simulink model "Copy_of_htx_estimator"  (R2024b)
settings: Solver=FixedStepAuto  StartTime=0.0  StopTime=10.0  RelTol=1e-3
undefined symbols (not defined in the file): dspblkCoreblockFVToolHelper, gcbh
libraries: simulink_extras x1
settings Model: Creator=lukec  LastModifiedBy=lukec
settings OptimizationCC: DefaultParameterBehavior=Inlined  EnhancedBackFolding=on  PassReuseOutputArgsAs=Individual arguments  ZeroExternalMemoryAtStartup=off  ZeroInternalMemoryAtStartup=off  OptimizeBlockOrder=speed  DifferentSizesBufferReuse=on  OptimizationCustomize=off  EfficientTunableParamExpr=on
settings DebuggingCC: ParameterTunabilityLossMsg=error
settings HardwareCC: ProdBitPerPointer=32  ProdBitPerSizeT=32  ProdBitPerPtrDiffT=32  ProdLargestAtomicInteger=Long  ProdLargestAtomicFloat=Double  ProdWordSize=32  ProdHWDeviceType=ARM Compatible->ARM Cortex-M
settings SFSimCC: MATLABDynamicMemAlloc=off
settings RTWCC: Description=Embedded Coder  SystemTargetFile=ert.tlc  GenCodeOnly=on  PackageGeneratedCodeAndArtifacts=on  TemplateMakefile=ert_default_tmf  Toolchain=CMake  TargetLang=C++
settings CodeAppCC: ForceParamTrailComments=on  IgnoreCustomStorageClasses=off  MaxIdLength=255  OperatorAnnotations=on  SimulinkDataObjDesc=on  SFDataObjDesc=on  InsertBlockDesc=on
settings ERTTargetCC: TargetLangStandard=C++17 (ISO)  CodeInterfacePackaging=C++ class  RootIOFormat=Structure reference  ERTCustomFileTemplate=example_file_process.tlc  ArrayContainerType=std::array

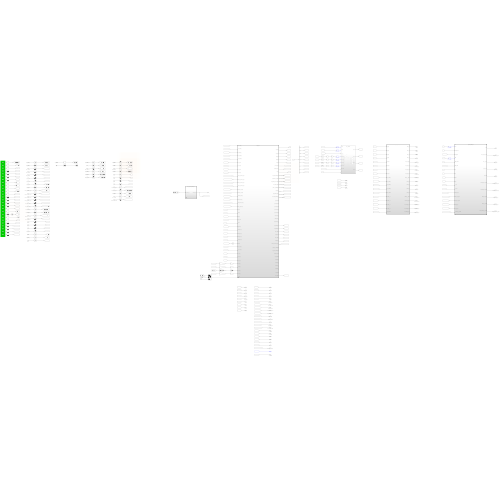
[thumbnail: Simulink's stored preview of the top-level diagram]
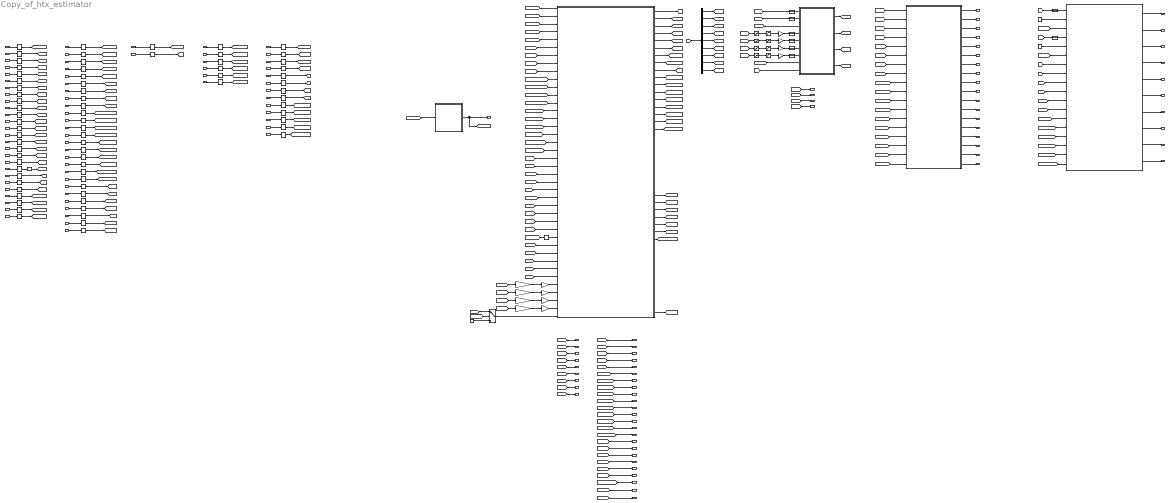
== system Copy_of_htx_estimator ==
  note: non-param-inputs
  steer_sensor_raw : Inport
  ax_m_s2 : Inport  Port=2
  ay_m_s2 : Inport  Port=3
  loadcell_fl : Inport  Port=4
  loadcell_fr : Inport  Port=5
  loadcell_rl : Inport  Port=6
  loadcell_rr : Inport  Port=7
  torq_Nm_fl : Inport  Port=8
  torq_Nm_fr : Inport  Port=9
  torq_Nm_rl : Inport  Port=10
  torq_Nm_rr : Inport  Port=11
  motor_rpm_fl : Inport  Port=12
  motor_rpm_fr : Inport  Port=13
  motor_rpm_rl : Inport  Port=14
  motor_rpm_rr : Inport  Port=15
  vx_raw_m_s : Inport  Port=16
  vy_raw_m_s : Inport  Port=17
  ins_vel_u : Inport  Port=18
  ins_mode : Inport  Port=19
  accel : Inport  Port=20
  brake : Inport  Port=21
  wz_rad_s : Inport  Port=22
  motor_temp_C_fl : Inport  Port=23
  motor_temp_C_fr : Inport  Port=24
  motor_temp_C_rl : Inport  Port=25
  motor_temp_C_rr : Inport  Port=26
  proc_vx_std_m_s : Inport  Port=27
  proc_vy_std_m_s : Inport  Port=28
  proc_r_std_deg_s : Inport  Port=29
  proc_ax_std_m_s2 : Inport  Port=30
  proc_ay_std_m_s2 : Inport  Port=31
  proc_sr_fl_std : Inport  Port=32
  proc_sr_fr_std : Inport  Port=33
  proc_sr_rl_std : Inport  Port=34
  proc_sr_rr_std : Inport  Port=35
  meas_ins_vx_mode1_std_m_s : Inport  Port=36
  meas_ins_vy_mode1_std_m_s : Inport  Port=37
  meas_ins_vx_mode2_std_m_s : Inport  Port=38
  meas_ins_vy_mode2_std_m_s : Inport  Port=39
  meas_imu_ax_std_m_s2 : Inport  Port=40
  meas_imu_ay_std_m_s2 : Inport  Port=41
  meas_imu_r_std_deg_s : Inport  Port=42
  meas_wss_std_deg_s : Inport  Port=43
  meas_pseudo_vx_std_m_s : Inport  Port=44
  meas_vy_gate_std_m_s : Inport  Port=45
  chi_ins_vx : Inport  Port=46
  chi_ins_vy : Inport  Port=47
  chi_imu_r : Inport  Port=48
  chi_imu_accel : Inport  Port=49
  chi_wss : Inport  Port=50
  chi_pseudo_vx : Inport  Port=51
  fz_meas_alpha : Inport  Port=52
  m_kg : Inport  Port=53
  amk_eff_modifier_fl : Inport  Port=54
  amk_eff_modifier_fr : Inport  Port=55
  amk_eff_modifier_rl : Inport  Port=56
  amk_eff_modifier_rr : Inport  Port=57
  global_eff_modifier : Inport  Port=58
  brake_eff_modifier : Inport  Port=59
  accel_deadzone : Inport  Port=60
  accel_gamma : Inport  Port=61
  brake_deadzone : Inport  Port=62
  brake_gamma : Inport  Port=63
  a_off : Inport  Port=64
  a_on : Inport  Port=65
  b_start : Inport  Port=66
  b_full : Inport  Port=67
  drive_motor_torq_lim : Inport  Port=68
  regen_motor_torq_lim : Inport  Port=69
  motor_rpm_lim : Inport  Port=70
  elec_p_lim_kW : Inport  Port=71
  per_motor_elec_p_lim_kW : Inport  Port=72
  use_ins : Inport  Port=73
  1-D Lookup Table : Lookup_n-D  NumberOfTableDimensions=1  BreakpointsForDimension1=|  Table=|  ExtrapMethod=Clip  InternalRulePriority=Speed  RndMeth=Simplest
      BreakpointsForDimension1=|
      | [159
      | 845
      | 1004
      | 1093
      | 1233
      | 1645
      | 1875
      | 2150
      | 2260]
      Table=|
      | [0
      | 87.3
      | 107.7
      | 120.1
      | 139.7
      | 193.3
      | 230.4
      | 269.1
      | 282.5]
  1-D Lookup Table1 : Lookup_n-D  NumberOfTableDimensions=1  BreakpointsForDimension1=|  Table=|  ExtrapMethod=Clip  InternalRulePriority=Speed  RndMeth=Simplest
      BreakpointsForDimension1=|
      | [191
      | 984
      | 1101
      | 1186
      | 1323
      | 1730
      | 1962
      | 2150
      | 2350
      | ]
      Table=|
      | [0
      | 102.4
      | 116.4
      | 128.2
      | 148.6
      | 198.5
      | 236.2
      | 260.2
      | 289.2
      | ]
  1-D Lookup Table2 : Lookup_n-D  NumberOfTableDimensions=1  BreakpointsForDimension1=|  Table=|  ExtrapMethod=Clip  InternalRulePriority=Speed  RndMeth=Simplest
      BreakpointsForDimension1=|
      | [223
      | 1017
      | 1069
      | 1193
      | 1260
      | 1730
      | 1992
      | 2170
      | 2310
      | ]
      Table=|
      | [0
      | 112.9
      | 117.6
      | 135.2
      | 146.8
      | 213.3
      | 250.6
      | 276.9
      | 296.5
      | ]
  1-D Lookup Table3 : Lookup_n-D  NumberOfTableDimensions=1  BreakpointsForDimension1=|  Table=|  ExtrapMethod=Clip  InternalRulePriority=Speed  RndMeth=Simplest
      BreakpointsForDimension1=|
      | [219
      | 908
      | 1006
      | 1134
      | 1180
      | 1685
      | 1935
      | 2093
      | 2240
      | ]
      Table=|
      | [0
      | 98.9
      | 110.4
      | 128.8
      | 137.2
      | 209.7
      | 242.8
      | 268.2
      | 288.5
      | ]
  Constant : Constant  Value=0
  Constant1 : Constant  Value=0
  Constant2 : Constant  Value=0
  Degrees to Radians : simulink_extras/Transformations/Degrees to Radians
  Demux : Demux  Outputs=9
  Floor : Rounding
  Gain{,2,4,6} (4 alike) : Gain  Gain=0.1047197551196598
  Gain{1,3,5,7} (4 alike) : Gain  Gain=1/11.83
  Gain{8..11} (4 alike) : Gain  Gain=4.4482
  Model : ModelReference  ModelNameDialog=htx_wheel_steer_estimator_base.slx  SimulationMode=Normal  ModelReferenceVersion=1.9
  Model1 : ModelReference  ModelNameDialog=htx_amk_eff_estimator_base.slx  SimulationMode=Normal  ModelReferenceVersion=1.36
  Model2 : ModelReference  ModelNameDialog=htx_intent_estimator_base.slx  SimulationMode=Normal  ModelReferenceVersion=1.15
  Model6 : ModelReference  ModelNameDialog=htx_ekf_base.slx  SimulationMode=Normal  ModelReferenceVersion=1.26
      settings: PortSchema="{\"entries\":[{\"content\":{\"sides\":[{\"content\":{\"connectorIds\":[\"In1\",\"In2\",\"In3\",\"In4\",\"In5\",\"In6\",\"In7\",\"In8\",\"In9\",\"In10\",\"In11\",\"In12\",\"In13\",\"In14\",\"In15\",\"In16\",\"In17\",\"In18\",\"In19\",\"In20\",\"In21\",\"In22\",\"In23\",\"In24\",\"In40\",\"In25\",\"In26\",\"In27\",\"In28\",\"In29\",\"In30\",\"In31\",\"In32\",\"In33\",\"In34\",\"In35\",\"In36\",\"In37\",\"In38\",\"In39\"]},\"type\":\"ConnectorPlacement.EquallySpacedRectSide\",\"uuid\":\"bb5109ea-6939-45c2-a357-a710596eeb4b\"},{\"content\":{\"connectorIds\":[\"Out1\",\"Out2\",\"Out3\",\"Out4\",\"Out5\",\"Out6\",\"Out7\",\"Out8\",\"Out9\",\"Out10\",\"Out11\",\"Out12\",\"Out13\",\"Out14\",\"Out15\",\"Out16\",\"Out17\",\"Out18\",\"Out19\",\"Out20\",\"Out21\",\"Out22\",\"Out23\",\"Out24\",\"Out25\",\"Out26\",\"Out27\",\"Out28\",\"Out29\",\"Out30\",\"Out31\",\"Out32\",\"Out33\",\"Out34\",\"Out35\",\"Out36\",\"Out37\",\"Out38\",\"Out39\",\"Out40\",\"Out41\",\"Out42\"],\"side\":\"RIGHT\"},\"type\":\"ConnectorPlacement.EquallySpacedRectSide\",\"uuid\":\"76f86590-693a-4540-9c0b-c0cd03bb8a5c\"},{\"content\":{\"side\":\"TOP\"},\"type\":\"ConnectorPlacement.EquallySpacedRectSide\",\"uuid\":\"14cceb79-494c-4b5e-a97a-eec243580695\"}]},\"type\":\"ConnectorPlacement.EquallySpacedConnector\",\"uuid\":\"129f1803-a8f8-4413-b20a-49775fdc7b41\"}],\"packageUris\":[\"http://schema.mathworks.com/mf0/Connector/R2020b\"],\"version\":\"1.0\"}"
  Rate Transition{,1..72} (73 alike) : RateTransition  OutPortSampleTime=0.004
  Saturation{,1..3} (4 alike) : Saturate  UpperLimit=350  LowerLimit=0
  Subsystem : Subsystem  ReferencedSubsystem=htx_fz_estimator
  Switch : Switch  Criteria=u2 > Threshold  SaturateOnIntegerOverflow=off  InputSameDT=off
  low-pass_0.035 {1..8} (8 alike) : DiscreteTransferFcn  LoadFcn=dspblkCoreblockFVToolHelper(gcbh,'load');  Numerator=[0, 0.1143]  Denominator=[1, -0.8857]
      settings: CopyFcn=dspblkCoreblockFVToolHelper(gcbh,'copy');  DeleteFcn=dspblkCoreblockFVToolHelper(gcbh,'close');  ModelCloseFcn=dspblkCoreblockFVToolHelper(gcbh,'close');  PreSaveFcn=dspblkCoreblockFVToolHelper(gcbh,'presave');  PostSaveFcn=dspblkCoreblockFVToolHelper(gcbh,'postsave');  CloseFcn=dspblkCoreblockFVToolHelper(gcbh,'close');
  wheel_steer_deg : Outport
  ekf_vx_m_s : Outport  Port=2
  ekf_vy_m_s : Outport  Port=3
  ekf_r_rad_s : Outport  Port=4
  ekf_ax_m_s2 : Outport  Port=5
  ekf_ay_m_s2 : Outport  Port=6
  ekf_sr_fl : Outport  Port=7
  ekf_sr_fr : Outport  Port=8
  ekf_sr_rl : Outport  Port=9
  ekf_sr_rr : Outport  Port=10
  ins_vx_fault : Outport  Port=11
  ins_vy_fault : Outport  Port=12
  imu_r_fault : Outport  Port=13
  imu_a_fault : Outport  Port=14
  wss_fault : Outport  Port=15
  pseudo_vx_fault : Outport  Port=16
  use_pseudo_vx_flag : Outport  Port=17
  ins_supervisor_mode : Outport  Port=18
  ins_supervisor_fail_count : Outport  Port=19
  ins_supervisor_good_count : Outport  Port=20
  ins_reports_valid : Outport  Port=21
  pseudo_vx_available : Outport  Port=22
  use_ins_dbg : Outport  Port=23
  ins_vx_update_used : Outport  Port=24
  ins_low_speed_override : Outport  Port=25
  spin_detected : Outport  Port=26
  lock_detected : Outport  Port=27
  spin_front : Outport  Port=28
  spin_rear : Outport  Port=29
  lock_front : Outport  Port=30
  lock_rear : Outport  Port=31
  decouple_wss_from_vxvy : Outport  Port=32
  fz_est_N_fl : Outport  Port=33
  fz_est_N_fr : Outport  Port=34
  fz_est_N_rl : Outport  Port=35
  fz_est_N_rr : Outport  Port=36
  amk_eff_fl : Outport  Port=37
  amk_eff_fr : Outport  Port=38
  amk_eff_rl : Outport  Port=39
  amk_eff_rr : Outport  Port=40
  amk_elec_p_W_fl : Outport  Port=41
  amk_elec_p_W_fr : Outport  Port=42
  amk_elec_p_W_rl : Outport  Port=43
  amk_elec_p_W_rr : Outport  Port=44
  amk_elec_p_kW_tot : Outport  Port=45
  global_eff_fl : Outport  Port=46
  global_eff_fr : Outport  Port=47
  global_eff_rl : Outport  Port=48
  global_eff_rr : Outport  Port=49
  global_elec_p_kW_tot : Outport  Port=50
  motor_heat_gen_W_fl : Outport  Port=51
  motor_heat_gen_W_fr : Outport  Port=52
  motor_heat_gen_W_rl : Outport  Port=53
  motor_heat_gen_W_rr : Outport  Port=54
  intent : Outport  Port=55
  max_tot_motor_torq_Nm : Outport  Port=56
  des_wz_rad_s : Outport  Port=57
  w_z_error_rad_s : Outport  Port=58
  des_Mz_Nm : Outport  Port=59
  intent_drive_motor_torq_lim : Outport  Port=60
  intent_regen_motor_torq_lim : Outport  Port=61
  intent_motor_rpm_lim : Outport  Port=62
  intent_elec_p_lim_kW : Outport  Port=63
  intent_per_motor_elec_p_lim_kW : Outport  Port=64
  intent_use_ins : Outport  Port=65
  ins_state_dbg : Outport  Port=66
  wires:
  ax_m_s2/1 -> Rate Transition2/1
  motor_temp_C_fl/1 -> Rate Transition1/1
  motor_temp_C_rr/1 -> Rate Transition58/1
  torq_Nm_fr/1 -> Rate Transition9/1
  Rate Transition58/1 -> [motor_temp_C_rr]
  Rate Transition11/1 -> [torq_Nm_rr]
  Rate Transition22/1 -> [accel]
  Rate Transition/1 -> [steer_sensor_raw]
  Rate Transition13/1 -> Floor/1
  vy_raw_m_s/1 -> Rate Transition19/1
  loadcell_rl/1 -> Rate Transition6/1
  ins_vel_u/1 -> Rate Transition12/1
  Rate Transition3/1 -> [imu_ay_m_s2]
  Rate Transition18/1 -> [ins_vx_m_s]
  Rate Transition10/1 -> [torq_Nm_rl]
  Rate Transition4/1 -> [loadcell_fl]
  Rate Transition12/1 -> [ins_vel_u]
  Rate Transition59/1 -> [motor_temp_C_fr]
  motor_temp_C_rl/1 -> Rate Transition57/1
  loadcell_fl/1 -> Rate Transition4/1
  motor_rpm_rr/1 -> Rate Transition17/1
  brake/1 -> Rate Transition20/1
  steer_sensor_raw/1 -> Rate Transition/1
  vx_raw_m_s/1 -> Rate Transition18/1
  Rate Transition14/1 -> [motor_rpm_fl]
  Rate Transition7/1 -> [loadcell_rr]
  wz_rad_s/1 -> Rate Transition21/1
  Rate Transition5/1 -> [loadcell_fr]
  Rate Transition2/1 -> [imu_ax_m_s2]
  ins_mode/1 -> Rate Transition13/1
  Rate Transition17/1 -> [motor_rpm_rr]
  Rate Transition9/1 -> [torq_Nm_fr]
  accel/1 -> Rate Transition22/1
  torq_Nm_rl/1 -> Rate Transition10/1
  Rate Transition6/1 -> [loadcell_rl]
  motor_rpm_rl/1 -> Rate Transition16/1
  motor_rpm_fl/1 -> Rate Transition14/1
  motor_rpm_fr/1 -> Rate Transition15/1
  Rate Transition16/1 -> [motor_rpm_rl]
  Rate Transition19/1 -> [ins_vy_m_s]
  Rate Transition20/1 -> [brake]
  torq_Nm_rr/1 -> Rate Transition11/1
  loadcell_rr/1 -> Rate Transition7/1
  Rate Transition8/1 -> [torq_Nm_fl]
  Rate Transition15/1 -> [motor_rpm_fr]
  Rate Transition57/1 -> [motor_temp_C_rl]
  Rate Transition1/1 -> [motor_temp_C_fl]
  torq_Nm_fl/1 -> Rate Transition8/1
  motor_temp_C_fr/1 -> Rate Transition59/1
  loadcell_fr/1 -> Rate Transition5/1
  ay_m_s2/1 -> Rate Transition3/1
  Rate Transition21/1 -> [imu_r_rad_s]
  [steer_sensor_raw] -> Model/1
  Model/1 -> wheel_steer_deg/1, [wheel_steer_deg]
  low-pass_0.035 5/1 -> Subsystem/1
  [imu_ax_m_s2] -> low-pass_0.035 5/1
  low-pass_0.035 6/1 -> Subsystem/2
  [imu_ay_m_s2] -> low-pass_0.035 6/1
  [loadcell_fr] -> 1-D Lookup Table1/1
  [loadcell_rl] -> 1-D Lookup Table2/1
  [loadcell_rr] -> 1-D Lookup Table3/1
  1-D Lookup Table/1 -> Saturation/1
  low-pass_0.035 3/1 -> Subsystem/4
  1-D Lookup Table1/1 -> Saturation1/1
  low-pass_0.035 2/1 -> Subsystem/6
  low-pass_0.035 4/1 -> Subsystem/7
  low-pass_0.035 1/1 -> Subsystem/5
  1-D Lookup Table2/1 -> Saturation2/1
  1-D Lookup Table3/1 -> Saturation3/1
  Subsystem/1 -> [fz_est_N_fl]
  Subsystem/2 -> [fz_est_N_fr]
  Subsystem/3 -> [fz_est_N_rl]
  Subsystem/4 -> [fz_est_N_rr]
  [torq_Nm_fl] -> Model6/25
  [torq_Nm_fr] -> Model6/26
  [torq_Nm_rl] -> Model6/27
  [torq_Nm_rr] -> Model6/28
  [wheel_steer_deg] -> Degrees to Radians/1
  Degrees to Radians/1 -> Model6/29
  [ins_vx_m_s] -> Model6/30
  [ins_vy_m_s] -> Model6/31
  [imu_r_rad_s] -> Model6/32
  [imu_ax_m_s2] -> Model6/33
  [imu_ay_m_s2] -> Model6/34
  [motor_rpm_fl] -> Gain/1
  Gain/1 -> Gain1/1
  Gain1/1 -> Model6/35
  Gain3/1 -> Model6/36
  [motor_rpm_fr] -> Gain2/1
  [motor_rpm_rl] -> Gain4/1
  Gain5/1 -> Model6/37
  Gain7/1 -> Model6/38
  [motor_rpm_rr] -> Gain6/1
  Model6/1 -> [x]  "x"
  Model6/2 -> [ins_vx_fault]
  Model6/3 -> [ins_vy_fault]
  Model6/4 -> [imu_r_fault]
  Model6/5 -> [imu_a_fault]
  Model6/6 -> [wss_fault]
  Model6/7 -> [pseudo_vx_fault]
  Model6/8 -> [use_pseudo_vx_flag]
  Model6/9 -> [P_diag]
  Model6/10 -> [ins_supervisor_mode]  "ins_supervisor_mode_dbg"
  Model6/11 -> [ins_supervisor_fail_count]  "ins_supervisor_fail_count_dbg"
  Model6/12 -> [ins_supervisor_good_count]  "ins_supervisor_good_count_dbg"
  Model6/13 -> [ins_resports_valid]  "ins_reports_valid_dbg"
  Model6/14 -> [pseudo_vx_available]  "pseudo_vx_available_dbg"
  Model6/15 -> [use_ins_dbg]  "use_ins_dbg"
  Model6/16 -> [ins_vx_update_used]  "ins_vx_update_used_dbg"
  Model6/17 -> [ins_low_speed_override]  "ins_low_speed_override_dbg"
  Model6/26 -> [spin_detected]
  Model6/27 -> [lock_detected]
  Model6/28 -> [spin_front]
  Model6/29 -> [spin_rear]
  Model6/30 -> [lock_front]
  Model6/31 -> [lock_rear]
  Model6/32 -> [decouple_wss_from_vxvy]
  [x] -> Demux/1  "x"
  Demux/1 -> [ekf_vx_m_s]  "vx_m_s"
  Demux/2 -> [ekf_vy_m_s]  "vy_m_s"
  Demux/3 -> [ekf_r_rad_s]  "r_rad_s"
  Demux/4 -> [ekf_ax_m_s2]  "ax_m_s2"
  Demux/5 -> [ekf_ay_m_s2]  "ay_m_s2"
  Demux/6 -> [ekf_sr_fl]  "sr_fl"
  Demux/7 -> [ekf_sr_fr]  "sr_fr"
  Demux/8 -> [ekf_sr_rl]  "sr_rl"
  Demux/9 -> [ekf_sr_rr]  "sr_rr"
  [ekf_vx_m_s] -> Subsystem/3
  [torq_Nm_fl] -> Model1/1
  [torq_Nm_fr] -> Model1/2
  [torq_Nm_rl] -> Model1/3
  [torq_Nm_rr] -> Model1/4
  [motor_rpm_fl] -> Model1/5
  [motor_rpm_fr] -> Model1/6
  [motor_rpm_rl] -> Model1/7
  [motor_rpm_rr] -> Model1/8
  [motor_temp_C_fl] -> Model1/14
  [motor_temp_C_rr] -> Model1/17
  [motor_temp_C_rl] -> Model1/16
  [motor_temp_C_fr] -> Model1/15
  [ekf_vx_m_s] -> ekf_vx_m_s/1
  [ekf_vy_m_s] -> ekf_vy_m_s/1
  [ekf_r_rad_s] -> ekf_r_rad_s/1
  [ekf_ax_m_s2] -> ekf_ax_m_s2/1
  [ekf_ay_m_s2] -> ekf_ay_m_s2/1
  [ekf_sr_fl] -> ekf_sr_fl/1
  [ekf_sr_fr] -> ekf_sr_fr/1
  [ekf_sr_rl] -> ekf_sr_rl/1
  [ekf_sr_rr] -> ekf_sr_rr/1
  [ins_vx_fault] -> ins_vx_fault/1
  [ins_vy_fault] -> ins_vy_fault/1
  [imu_r_fault] -> imu_r_fault/1
  [pseudo_vx_fault] -> pseudo_vx_fault/1
  [wss_fault] -> wss_fault/1
  [imu_a_fault] -> imu_a_fault/1
  [use_pseudo_vx_flag] -> use_pseudo_vx_flag/1
  [ins_supervisor_mode] -> ins_supervisor_mode/1
  [ins_supervisor_fail_count] -> ins_supervisor_fail_count/1
  [ins_supervisor_good_count] -> ins_supervisor_good_count/1
  [ins_resports_valid] -> ins_reports_valid/1
  [pseudo_vx_available] -> pseudo_vx_available/1
  [use_ins_dbg] -> use_ins_dbg/1
  [ins_vx_update_used] -> ins_vx_update_used/1
  [ins_low_speed_override] -> ins_low_speed_override/1
  [spin_detected] -> spin_detected/1
  [lock_detected] -> lock_detected/1
  [spin_front] -> spin_front/1
  [spin_rear] -> spin_rear/1
  [lock_front] -> lock_front/1
  [lock_rear] -> lock_rear/1
  [decouple_wss_from_vxvy] -> decouple_wss_from_vxvy/1
  [fz_est_N_fl] -> fz_est_N_fl/1
  [fz_est_N_fr] -> fz_est_N_fr/1
  [fz_est_N_rl] -> fz_est_N_rl/1
  [fz_est_N_rr] -> fz_est_N_rr/1
  Model1/1 -> amk_eff_fl/1
  Model1/2 -> amk_eff_fr/1
  Model1/3 -> amk_eff_rl/1
  Model1/4 -> amk_eff_rr/1
  Model1/5 -> amk_elec_p_W_fl/1
  Model1/6 -> amk_elec_p_W_fr/1
  Model1/7 -> amk_elec_p_W_rl/1
  Model1/8 -> amk_elec_p_W_rr/1
  Model1/9 -> amk_elec_p_kW_tot/1
  Model1/10 -> global_eff_fl/1
  Model1/11 -> global_eff_fr/1
  Model1/12 -> global_eff_rl/1
  Model1/13 -> global_eff_rr/1
  Model1/14 -> global_elec_p_kW_tot/1
  Model1/15 -> motor_heat_gen_W_fl/1
  Model1/16 -> motor_heat_gen_W_fr/1
  Model1/17 -> motor_heat_gen_W_rl/1
  Model1/18 -> motor_heat_gen_W_rr/1
  [accel] -> low-pass_0.035 8/1
  [brake] -> low-pass_0.035 7/1
  [ekf_vx_m_s] -> Model2/11
  [ekf_r_rad_s] -> Model2/12
  [wheel_steer_deg] -> Model2/13
  Model2/1 -> intent/1
  Model2/2 -> max_tot_motor_torq_Nm/1
  Model2/3 -> des_wz_rad_s/1
  Model2/4 -> w_z_error_rad_s/1
  Model2/6 -> intent_drive_motor_torq_lim/1
  Model2/7 -> intent_regen_motor_torq_lim/1
  Model2/8 -> intent_motor_rpm_lim/1
  Model2/9 -> intent_elec_p_lim_kW/1
  Model2/10 -> intent_per_motor_elec_p_lim_kW/1
  [chi_pseudo_vx] -> Model6/40
  [chi_wss] -> Model6/24
  [chi_imu_accel] -> Model6/23
  [chi_imu_r] -> Model6/22
  [chi_ins_vy] -> Model6/21
  [chi_ins_vx] -> Model6/20
  [meas_vy_gate_std_m_s] -> Model6/19
  [meas_pseudo_vx_std_m_s] -> Model6/18
  [meas_wss_std_deg_s] -> Model6/17
  [meas_imu_r_std_deg_s] -> Model6/16
  [meas_imu_ax_std_m_s2] -> Model6/14
  [meas_imu_ay_std_m_s2] -> Model6/15
  [meas_ins_vy_mode2_std_m_s] -> Model6/13
  [meas_ins_vx_mode2_std_m_s] -> Model6/12
  [meas_ins_vx_mode1_std_m_s] -> Model6/10
  [meas_ins_vy_mode1_std_m_s] -> Model6/11
  [proc_sr_rr_std] -> Model6/9
  [proc_sr_fl_std] -> Model6/6
  [proc_sr_fr_std] -> Model6/7
  [proc_sr_rl_std] -> Model6/8
  [proc_vx_std_m_s] -> Model6/1
  [proc_vy_std_m_s] -> Model6/2
  [proc_r_std_deg_s] -> Model6/3
  [proc_ax_std_m_s2] -> Model6/4
  [proc_ay_std_m_s2] -> Model6/5
  Rate Transition23/1 -> [proc_vx_std_m_s]
  proc_vx_std_m_s/1 -> Rate Transition23/1
  proc_vy_std_m_s/1 -> Rate Transition25/1
  proc_ax_std_m_s2/1 -> Rate Transition26/1
  proc_r_std_deg_s/1 -> Rate Transition24/1
  Rate Transition24/1 -> [proc_r_std_deg_s]
  Rate Transition25/1 -> [proc_vy_std_m_s]
  Rate Transition26/1 -> [proc_ax_std_m_s2]
  proc_sr_fr_std/1 -> Rate Transition28/1
  proc_sr_rl_std/1 -> Rate Transition30/1
  proc_sr_fl_std/1 -> Rate Transition29/1
  proc_ay_std_m_s2/1 -> Rate Transition27/1
  proc_sr_rr_std/1 -> Rate Transition31/1
  meas_ins_vx_mode1_std_m_s/1 -> Rate Transition33/1
  meas_ins_vx_mode2_std_m_s/1 -> Rate Transition34/1
  meas_ins_vy_mode1_std_m_s/1 -> Rate Transition32/1
  meas_imu_ay_std_m_s2/1 -> Rate Transition36/1
  meas_imu_r_std_deg_s/1 -> Rate Transition38/1
  meas_imu_ax_std_m_s2/1 -> Rate Transition37/1
  meas_ins_vy_mode2_std_m_s/1 -> Rate Transition35/1
  meas_wss_std_deg_s/1 -> Rate Transition39/1
  meas_pseudo_vx_std_m_s/1 -> Rate Transition41/1
  chi_ins_vx/1 -> Rate Transition42/1
  meas_vy_gate_std_m_s/1 -> Rate Transition40/1
  chi_imu_accel/1 -> Rate Transition44/1
  chi_wss/1 -> Rate Transition46/1
  chi_imu_r/1 -> Rate Transition45/1
  chi_ins_vy/1 -> Rate Transition43/1
  chi_pseudo_vx/1 -> Rate Transition47/1
  Rate Transition47/1 -> [chi_pseudo_vx]
  Rate Transition46/1 -> [chi_wss]
  Rate Transition44/1 -> [chi_imu_accel]
  Rate Transition45/1 -> [chi_imu_r]
  Rate Transition43/1 -> [chi_ins_vy]
  Rate Transition42/1 -> [chi_ins_vx]
  Rate Transition40/1 -> [meas_vy_gate_std_m_s]
  Rate Transition41/1 -> [meas_pseudo_vx_std_m_s]
  Rate Transition33/1 -> [meas_ins_vx_mode1_std_m_s]
  Rate Transition32/1 -> [meas_ins_vy_mode1_std_m_s]
  Rate Transition34/1 -> [meas_ins_vx_mode2_std_m_s]
  Rate Transition35/1 -> [meas_ins_vy_mode2_std_m_s]
  Rate Transition37/1 -> [meas_imu_ax_std_m_s2]
  Rate Transition36/1 -> [meas_imu_ay_std_m_s2]
  Rate Transition38/1 -> [meas_imu_r_std_deg_s]
  Rate Transition39/1 -> [meas_wss_std_deg_s]
  Rate Transition27/1 -> [proc_ay_std_m_s2]
  Rate Transition29/1 -> [proc_sr_fl_std]
  Rate Transition28/1 -> [proc_sr_fr_std]
  Rate Transition30/1 -> [proc_sr_rl_std]
  Rate Transition31/1 -> [proc_sr_rr_std]
  [fz_meas_alpha] -> Subsystem/8
  [m_kg] -> Subsystem/9
  fz_meas_alpha/1 -> Rate Transition48/1
  Rate Transition48/1 -> [fz_meas_alpha]
  m_kg/1 -> Rate Transition49/1
  Rate Transition49/1 -> [m_kg]
  brake_eff_modifier/1 -> Rate Transition62/1
  Rate Transition54/1 -> [amk_eff_modifier_rl]
  amk_eff_modifier_fr/1 -> Rate Transition53/1
  amk_eff_modifier_rl/1 -> Rate Transition54/1
  Rate Transition55/1 -> [amk_eff_modifier_rr]
  amk_eff_modifier_rr/1 -> Rate Transition55/1
  Rate Transition62/1 -> [brake_eff_modifier]
  Rate Transition53/1 -> [amk_eff_modifier_fr]
  global_eff_modifier/1 -> Rate Transition56/1
  Rate Transition56/1 -> [global_eff_modifier]
  Rate Transition50/1 -> [amk_eff_modifier_fl]
  amk_eff_modifier_fl/1 -> Rate Transition50/1
  [amk_eff_modifier_fl] -> Model1/9
  [amk_eff_modifier_fr] -> Model1/10
  [amk_eff_modifier_rl] -> Model1/11
  [amk_eff_modifier_rr] -> Model1/12
  [global_eff_modifier] -> Model1/13
  [brake_eff_modifier] -> Model1/18
  Constant1/1 -> Model2/2
  [accel_gamma] -> Model2/3
  Constant2/1 -> Model2/5
  [brake_gamma] -> Model2/6
  [a_off] -> Model2/7
  [a_on] -> Model2/8
  [b_start] -> Model2/9
  [b_full] -> Model2/10
  [per_motor_elec_p_lim_kW] -> Model2/18
  [elec_p_lim_kW] -> Model2/17
  [motor_rpm_lim] -> Model2/16
  [regen_motor_torq_lim] -> Model2/15
  [drive_motor_torq_lim] -> Model2/14
  accel_deadzone/1 -> Rate Transition51/1
  accel_gamma/1 -> Rate Transition52/1
  brake_deadzone/1 -> Rate Transition60/1
  a_on/1 -> Rate Transition64/1
  brake_gamma/1 -> Rate Transition61/1
  a_off/1 -> Rate Transition63/1
  b_start/1 -> Rate Transition65/1
  b_full/1 -> Rate Transition66/1
  drive_motor_torq_lim/1 -> Rate Transition67/1
  elec_p_lim_kW/1 -> Rate Transition70/1
  regen_motor_torq_lim/1 -> Rate Transition68/1
  motor_rpm_lim/1 -> Rate Transition69/1
  per_motor_elec_p_lim_kW/1 -> Rate Transition71/1
  Rate Transition51/1 -> [accel_deadzone]
  Rate Transition52/1 -> [accel_gamma]
  Rate Transition60/1 -> [brake_deadzone]
  Rate Transition61/1 -> [brake_gamma]
  Rate Transition63/1 -> [a_off]
  Rate Transition64/1 -> [a_on]
  Rate Transition65/1 -> [b_start]
  Rate Transition66/1 -> [b_full]
  Rate Transition67/1 -> [drive_motor_torq_lim]
  Rate Transition68/1 -> [regen_motor_torq_lim]
  Rate Transition69/1 -> [motor_rpm_lim]
  Rate Transition70/1 -> [elec_p_lim_kW]
  Rate Transition71/1 -> [per_motor_elec_p_lim_kW]
  low-pass_0.035 8/1 -> Model2/1
  low-pass_0.035 7/1 -> Model2/4
  Model2/5 -> des_Mz_Nm/1
  use_ins/1 -> Rate Transition72/1
  Rate Transition72/1 -> [use_ins]
  [use_ins] -> Switch/2
  [ins_mode] -> Switch/1
  Constant/1 -> Switch/3
  Switch/1 -> Model6/39
  [use_ins] -> intent_use_ins/1
  Floor/1 -> [ins_mode]
  Gain8/1 -> low-pass_0.035 3/1
  Gain9/1 -> low-pass_0.035 1/1
  Gain10/1 -> low-pass_0.035 2/1
  Gain11/1 -> low-pass_0.035 4/1
  [loadcell_fl] -> 1-D Lookup Table/1
  Saturation/1 -> Gain8/1
  Saturation1/1 -> Gain9/1
  Saturation2/1 -> Gain10/1
  Saturation3/1 -> Gain11/1
  Model6/42 -> [ins_state_dbg]
  [ins_state_dbg] -> ins_state_dbg/1
  Gain2/1 -> Gain3/1
  Gain4/1 -> Gain5/1
  Gain6/1 -> Gain7/1
